simulink library "tqr"  (R2021b)
settings: Solver=VariableStepAuto  StartTime=0.0  StopTime=10.0  RelTol=1e-3
undefined symbols (not defined in the file or in its folder): ATQR_AltRDCActiveFEDUInc_X_pct, ATQR_AltRDCActiveFEDUInc_Y_enum, ATQR_AltRDCActiveFEDUTs_X_pct, ATQR_AltRDCActiveFEDUTs_Y_enum, ATQR_AltRDCActiveREDUInc_X_pct, ATQR_AltRDCActiveREDUInc_Y_enum, ATQR_AltRDCActiveREDUTs_X_pct, ATQR_AltRDCActiveREDUTs_Y_enum, ATQR_CreepFEDUTqIncSR_X_rpm, ATQR_CreepFEDUTqIncSR_Y_Nm, ATQR_CreepFEDUTs_X_rpm, ATQR_CreepFEDUTs_Y_Nm, ATQR_EcoTqFrIncGain_X_Nm, ATQR_EcoTqFrIncGain_Y_pct, ATQR_EcoTqRrIncGain_X_Nm, ATQR_EcoTqRrIncGain_Y_pct, ATQR_EL1FEDUTqDecSR_Y_Nm, ATQR_EL1FEDUTqIncSR_X_rpm, ATQR_EL1FEDUTqIncSR_Y_pct, ATQR_EL1FEDUTs_X_rpm, ATQR_EL1FEDUTs_Y_Nm, ATQR_EL1REDUTqDecSR_Y_Nm, ATQR_EL1REDUTs_Y_Nm, ATQR_FEDUEL1RegenTs_X_rpm, ATQR_FEDUTIPOutTs_X_rpm, ATQR_FrNegRateLimitIncN_X_rpm, ATQR_FrNegRateLimitIncN_Y_Nm, ATQR_FrPosRateLimitIncN_X_rpm, ATQR_FrPosRateLimitIncN_Y_Nm, ATQR_FShaftSpdTqLimCoe_X_rpm, ATQR_FTimerTqLimCoe_X_s, ATQR_FTqZeroTransUpBoundN_X_rpm, ATQR_NL1FEDUTqDecSR_Y_Nm, ATQR_NL1FEDUTqIncSR_X_rpm, ATQR_NL1FEDUTqIncSR_Y_pct, ATQR_NL1FEDUTs_X_rpm, ATQR_NL1FEDUTs_Y_Nm, ATQR_NL1REDUTqDecSR_Y_Nm, ATQR_NL1REDUTs_Y_Nm, ATQR_NormalTqFrIncGain_X_Nm, ATQR_NormalTqFrIncGain_Y_pct, ATQR_NormalTqRrIncGain_X_Nm, ATQR_NormalTqRrIncGain_Y_pct, ATQR_RrNegRateLimitIncN_X_rpm, ATQR_RrNegRateLimitIncN_Y_Nm, ATQR_RrPosRateLimitIncN_X_rpm, ATQR_RrPosRateLimitIncN_Y_Nm, ATQR_RShaftSpdTqLimCoe_X_rpm, ATQR_RTimerTqLimCoe_X_s, ATQR_SL1FEDUTqDecSR_Y_Nm, ATQR_SL1FEDUTqIncSR_X_rpm, ATQR_SL1FEDUTqIncSR_Y_pct, ATQR_SL1FEDUTs_X_rpm, ATQR_SL1FEDUTs_Y_Nm, ATQR_SL1REDUTqDecSR_Y_Nm, ATQR_SL1REDUTs_Y_Nm, ATQR_SportTqFrIncGain_X_Nm, ATQR_SportTqFrIncGain_Y_pct, ATQR_SportTqRrIncGain_X_Nm, ATQR_SportTqRrIncGain_Y_pct ... (+261)
libraries: hcu_lib x14, simulink x12, $bdroot x3
(part 7 of 9)

== system tqr/TQR/Determine Torque Request/TorqueArbitrament/TorqueSmooth/Front First order filter input tau map and determination/VTQR_SPORTFEDUTs_c/Invalid ==
  VTQR_FEDUWhlTqReqSmoothDelay_Nm : Inport
  VTQD_TqTargetShaftSpd_rpm : Inport  Port=2
  Action Port : ActionPort
  MTQR_SL1FEDUTs_Z_c : Lookup_n-D  BreakpointsForDimension1=ATQR_SL1FEDUTs_Y_Nm  BreakpointsForDimension2=ATQR_SL1FEDUTs_X_rpm  Table=MTQR_SL1FEDUTs_Z_c  ExtrapMethod=Clip  InternalRulePriority=Speed  RndMeth=Simplest  InputSameDT=on
      settings: InputPortMap=u0,u1
  VTQR_SL1FEDUTs_c : Outport
  wires:
  VTQR_FEDUWhlTqReqSmoothDelay_Nm/1 -> MTQR_SL1FEDUTs_Z_c/1
  VTQD_TqTargetShaftSpd_rpm/1 -> MTQR_SL1FEDUTs_Z_c/2
  MTQR_SL1FEDUTs_Z_c/1 -> VTQR_SL1FEDUTs_c/1

== system tqr/TQR/Determine Torque Request/TorqueArbitrament/TorqueSmooth/Front First order filter input tau map and determination/VTQR_SPORTFEDUTs_c/LV1 ==
  VTQR_FEDUWhlTqReqSmoothDelay_Nm : Inport
  VTQD_TqTargetShaftSpd_rpm : Inport  Port=2
  Action Port : ActionPort
  MTQR_SL1FEDUTs_Z_c : Lookup_n-D  BreakpointsForDimension1=ATQR_SL1FEDUTs_Y_Nm  BreakpointsForDimension2=ATQR_SL1FEDUTs_X_rpm  Table=MTQR_SL1FEDUTs_Z_c  ExtrapMethod=Clip  InternalRulePriority=Speed  RndMeth=Simplest  InputSameDT=on
      settings: InputPortMap=u0,u1
  VTQR_SL1FEDUTs_c : Outport
  wires:
  MTQR_SL1FEDUTs_Z_c/1 -> VTQR_SL1FEDUTs_c/1
  VTQD_TqTargetShaftSpd_rpm/1 -> MTQR_SL1FEDUTs_Z_c/2
  VTQR_FEDUWhlTqReqSmoothDelay_Nm/1 -> MTQR_SL1FEDUTs_Z_c/1

== system tqr/TQR/Determine Torque Request/TorqueArbitrament/TorqueSmooth/Front First order filter input tau map and determination/VTQR_SPORTFEDUTs_c/LV2 ==
  VTQR_FEDUWhlTqReqSmoothDelay_Nm : Inport
  VTQD_TqTargetShaftSpd_rpm : Inport  Port=2
  Action Port : ActionPort
  MTQR_SL2FEDUTs_Z_c : Lookup_n-D  BreakpointsForDimension1=ATQR_SL1FEDUTs_Y_Nm  BreakpointsForDimension2=ATQR_SL1FEDUTs_X_rpm  Table=MTQR_SL2FEDUTs_Z_c  ExtrapMethod=Clip  InternalRulePriority=Speed  RndMeth=Simplest  InputSameDT=on
      settings: InputPortMap=u0,u1
  VTQR_SL2FEDUTs_c : Outport
  wires:
  VTQR_FEDUWhlTqReqSmoothDelay_Nm/1 -> MTQR_SL2FEDUTs_Z_c/1
  VTQD_TqTargetShaftSpd_rpm/1 -> MTQR_SL2FEDUTs_Z_c/2
  MTQR_SL2FEDUTs_Z_c/1 -> VTQR_SL2FEDUTs_c/1

== system tqr/TQR/Determine Torque Request/TorqueArbitrament/TorqueSmooth/Front First order filter input tau map and determination/VTQR_SPORTFEDUTs_c/LV3 ==
  VTQR_FEDUWhlTqReqSmoothDelay_Nm : Inport
  VTQD_TqTargetShaftSpd_rpm : Inport  Port=2
  Action Port : ActionPort
  MTQR_SL3FEDUTs_Z_c : Lookup_n-D  BreakpointsForDimension1=ATQR_SL1FEDUTs_Y_Nm  BreakpointsForDimension2=ATQR_SL1FEDUTs_X_rpm  Table=MTQR_SL3FEDUTs_Z_c  ExtrapMethod=Clip  InternalRulePriority=Speed  RndMeth=Simplest  InputSameDT=on
      settings: InputPortMap=u0,u1
  VTQR_SL3FEDUTs_c : Outport
  wires:
  VTQR_FEDUWhlTqReqSmoothDelay_Nm/1 -> MTQR_SL3FEDUTs_Z_c/1
  VTQD_TqTargetShaftSpd_rpm/1 -> MTQR_SL3FEDUTs_Z_c/2
  MTQR_SL3FEDUTs_Z_c/1 -> VTQR_SL3FEDUTs_c/1

== system tqr/TQR/Determine Torque Request/TorqueArbitrament/TorqueSmooth/Front First order filter input tau map and determination/VTQR_SPORTFEDUTs_c/LV4 ==
  VTQR_FEDUWhlTqReqSmoothDelay_Nm : Inport
  VTQD_TqTargetShaftSpd_rpm : Inport  Port=2
  Action Port : ActionPort
  MTQR_SL4FEDUTs_Z_c : Lookup_n-D  BreakpointsForDimension1=ATQR_SL1FEDUTs_Y_Nm  BreakpointsForDimension2=ATQR_SL1FEDUTs_X_rpm  Table=MTQR_SL4FEDUTs_Z_c  ExtrapMethod=Clip  InternalRulePriority=Speed  RndMeth=Simplest  InputSameDT=on
      settings: InputPortMap=u0,u1
  VTQR_SL4FEDUTs_c : Outport
  wires:
  VTQR_FEDUWhlTqReqSmoothDelay_Nm/1 -> MTQR_SL4FEDUTs_Z_c/1
  VTQD_TqTargetShaftSpd_rpm/1 -> MTQR_SL4FEDUTs_Z_c/2
  MTQR_SL4FEDUTs_Z_c/1 -> VTQR_SL4FEDUTs_c/1

== system tqr/TQR/Determine Torque Request/TorqueArbitrament/TorqueSmooth/Front First order filter input tau map and determination/VTQR_SPORTFEDUTs_c/LV5 ==
  VTQR_FEDUWhlTqReqSmoothDelay_Nm : Inport
  VTQD_TqTargetShaftSpd_rpm : Inport  Port=2
  Action Port : ActionPort
  MTQR_SL5FEDUTs_Z_c : Lookup_n-D  BreakpointsForDimension1=ATQR_SL1FEDUTs_Y_Nm  BreakpointsForDimension2=ATQR_SL1FEDUTs_X_rpm  Table=MTQR_SL5FEDUTs_Z_c  ExtrapMethod=Clip  InternalRulePriority=Speed  RndMeth=Simplest  InputSameDT=on
      settings: InputPortMap=u0,u1
  VTQR_SL5FEDUTs_c : Outport
  wires:
  VTQR_FEDUWhlTqReqSmoothDelay_Nm/1 -> MTQR_SL5FEDUTs_Z_c/1
  VTQD_TqTargetShaftSpd_rpm/1 -> MTQR_SL5FEDUTs_Z_c/2
  MTQR_SL5FEDUTs_Z_c/1 -> VTQR_SL5FEDUTs_c/1

== system tqr/TQR/Determine Torque Request/TorqueArbitrament/TorqueSmooth/Front First order filter input tau map and determination/VTQR_SPORTFEDUTs_c/OPD ==
  VTQR_FEDUWhlTqReqSmoothDelay_Nm : Inport
  VTQD_TqTargetShaftSpd_rpm : Inport  Port=2
  Action Port : ActionPort
  MTQR_SOPDFEDUTs_Z_c : Lookup_n-D  BreakpointsForDimension1=ATQR_SL1FEDUTs_Y_Nm  BreakpointsForDimension2=ATQR_SL1FEDUTs_X_rpm  Table=MTQR_SOPDFEDUTs_Z_c  ExtrapMethod=Clip  InternalRulePriority=Speed  RndMeth=Simplest  InputSameDT=on
      settings: InputPortMap=u0,u1
  VTQR_SOPDFEDUTs_c : Outport
  wires:
  VTQR_FEDUWhlTqReqSmoothDelay_Nm/1 -> MTQR_SOPDFEDUTs_Z_c/1
  VTQD_TqTargetShaftSpd_rpm/1 -> MTQR_SOPDFEDUTs_Z_c/2
  MTQR_SOPDFEDUTs_Z_c/1 -> VTQR_SOPDFEDUTs_c/1

== system tqr/TQR/Determine Torque Request/TorqueArbitrament/TorqueSmooth/Front wheel rate limit determination/Negative Rate limit Determination/VTQR_FrNegRateLimitDecE_Nm ==
  VTQD_TqTargetShaftSpd_rpm : Inport
  VTQR_FEDUWhlTqReqSmoothDelay_Nm : Inport  Port=2
  Action Port : ActionPort
  MTQR_FrNegRateLimitDecE_Z_Nm : Lookup_n-D  BreakpointsForDimension1=ATQR_FrNegRateLimitIncN_Y_Nm  BreakpointsForDimension2=ATQR_FrNegRateLimitIncN_X_rpm  Table=MTQR_FrNegRateLimitDecE_Z_Nm  ExtrapMethod=Clip  UseLastTableValue=on  InternalRulePriority=Speed  RndMeth=Simplest  InputSameDT=on
      settings: InputPortMap=u0,u1
  VTQR_FrNegRateLimitDecE_Nm : Outport
  wires:
  MTQR_FrNegRateLimitDecE_Z_Nm/1 -> VTQR_FrNegRateLimitDecE_Nm/1  "VTQR_FrNegRateLimitDecE_Nm"
  VTQR_FEDUWhlTqReqSmoothDelay_Nm/1 -> MTQR_FrNegRateLimitDecE_Z_Nm/1
  VTQD_TqTargetShaftSpd_rpm/1 -> MTQR_FrNegRateLimitDecE_Z_Nm/2

== system tqr/TQR/Determine Torque Request/TorqueArbitrament/TorqueSmooth/Front wheel rate limit determination/Negative Rate limit Determination/VTQR_FrNegRateLimitDecN_Nm ==
  VTQD_TqTargetShaftSpd_rpm : Inport
  VTQR_FEDUWhlTqReqSmoothDelay_Nm : Inport  Port=2
  Action Port : ActionPort
  MTQR_FrNegRateLimitDecN_Z_Nm : Lookup_n-D  BreakpointsForDimension1=ATQR_FrNegRateLimitIncN_Y_Nm  BreakpointsForDimension2=ATQR_FrNegRateLimitIncN_X_rpm  Table=MTQR_FrNegRateLimitDecN_Z_Nm  ExtrapMethod=Clip  UseLastTableValue=on  InternalRulePriority=Speed  RndMeth=Simplest  InputSameDT=on
      settings: InputPortMap=u0,u1
  VTQR_FrNegRateLimitDecN_Nm : Outport
  wires:
  MTQR_FrNegRateLimitDecN_Z_Nm/1 -> VTQR_FrNegRateLimitDecN_Nm/1  "VTQR_FrNegRateLimitDecN_Nm"
  VTQR_FEDUWhlTqReqSmoothDelay_Nm/1 -> MTQR_FrNegRateLimitDecN_Z_Nm/1
  VTQD_TqTargetShaftSpd_rpm/1 -> MTQR_FrNegRateLimitDecN_Z_Nm/2

== system tqr/TQR/Determine Torque Request/TorqueArbitrament/TorqueSmooth/Front wheel rate limit determination/Negative Rate limit Determination/VTQR_FrNegRateLimitDecS_Nm ==
  VTQD_TqTargetShaftSpd_rpm : Inport
  VTQR_FEDUWhlTqReqSmoothDelay_Nm : Inport  Port=2
  Action Port : ActionPort
  MTQR_FrNegRateLimitDecS_Z_Nm : Lookup_n-D  BreakpointsForDimension1=ATQR_FrNegRateLimitIncN_Y_Nm  BreakpointsForDimension2=ATQR_FrNegRateLimitIncN_X_rpm  Table=MTQR_FrNegRateLimitDecS_Z_Nm  ExtrapMethod=Clip  UseLastTableValue=on  InternalRulePriority=Speed  RndMeth=Simplest  InputSameDT=on
      settings: InputPortMap=u0,u1
  VTQR_FrNegRateLimitDecS_Nm : Outport
  wires:
  MTQR_FrNegRateLimitDecS_Z_Nm/1 -> VTQR_FrNegRateLimitDecS_Nm/1  "VTQR_FrNegRateLimitDecS_Nm"
  VTQD_TqTargetShaftSpd_rpm/1 -> MTQR_FrNegRateLimitDecS_Z_Nm/2
  VTQR_FEDUWhlTqReqSmoothDelay_Nm/1 -> MTQR_FrNegRateLimitDecS_Z_Nm/1

== system tqr/TQR/Determine Torque Request/TorqueArbitrament/TorqueSmooth/Front wheel rate limit determination/Negative Rate limit Determination/VTQR_FrNegRateLimitIncE_Nm ==
  VTQD_TqTargetShaftSpd_rpm : Inport
  VTQR_FEDUWhlTqReqSmoothDelay_Nm : Inport  Port=2
  Action Port : ActionPort
  MTQR_FrNegRateLimitIncE_Z_Nm : Lookup_n-D  BreakpointsForDimension1=ATQR_FrNegRateLimitIncN_Y_Nm  BreakpointsForDimension2=ATQR_FrNegRateLimitIncN_X_rpm  Table=MTQR_FrNegRateLimitIncE_Z_Nm  ExtrapMethod=Clip  UseLastTableValue=on  InternalRulePriority=Speed  RndMeth=Simplest  InputSameDT=on
      settings: InputPortMap=u0,u1
  VTQR_FrNegRateLimitIncE_Nm : Outport
  wires:
  MTQR_FrNegRateLimitIncE_Z_Nm/1 -> VTQR_FrNegRateLimitIncE_Nm/1  "VTQR_FrNegRateLimitIncE_Nm"
  VTQR_FEDUWhlTqReqSmoothDelay_Nm/1 -> MTQR_FrNegRateLimitIncE_Z_Nm/1
  VTQD_TqTargetShaftSpd_rpm/1 -> MTQR_FrNegRateLimitIncE_Z_Nm/2

== system tqr/TQR/Determine Torque Request/TorqueArbitrament/TorqueSmooth/Front wheel rate limit determination/Negative Rate limit Determination/VTQR_FrNegRateLimitIncN_Nm ==
  VTQD_TqTargetShaftSpd_rpm : Inport
  VTQR_FEDUWhlTqReqSmoothDelay_Nm : Inport  Port=2
  Action Port : ActionPort
  MTQR_FrNegRateLimitIncN_Z_Nm : Lookup_n-D  BreakpointsForDimension1=ATQR_FrNegRateLimitIncN_Y_Nm  BreakpointsForDimension2=ATQR_FrNegRateLimitIncN_X_rpm  Table=MTQR_FrNegRateLimitIncN_Z_Nm  ExtrapMethod=Clip  UseLastTableValue=on  InternalRulePriority=Speed  RndMeth=Simplest  InputSameDT=on
      settings: InputPortMap=u0,u1
  VTQR_FrNegRateLimitIncN_Nm : Outport
  wires:
  MTQR_FrNegRateLimitIncN_Z_Nm/1 -> VTQR_FrNegRateLimitIncN_Nm/1  "VTQR_FrNegRateLimitIncN_Nm"
  VTQR_FEDUWhlTqReqSmoothDelay_Nm/1 -> MTQR_FrNegRateLimitIncN_Z_Nm/1
  VTQD_TqTargetShaftSpd_rpm/1 -> MTQR_FrNegRateLimitIncN_Z_Nm/2

== system tqr/TQR/Determine Torque Request/TorqueArbitrament/TorqueSmooth/Front wheel rate limit determination/Negative Rate limit Determination/VTQR_FrNegRateLimitIncS_Nm ==
  VTQD_TqTargetShaftSpd_rpm : Inport
  VTQR_FEDUWhlTqReqSmoothDelay_Nm : Inport  Port=2
  Action Port : ActionPort
  MTQR_FrNegRateLimitIncS_Z_Nm : Lookup_n-D  BreakpointsForDimension1=ATQR_FrNegRateLimitIncN_Y_Nm  BreakpointsForDimension2=ATQR_FrNegRateLimitIncN_X_rpm  Table=MTQR_FrNegRateLimitIncS_Z_Nm  ExtrapMethod=Clip  UseLastTableValue=on  InternalRulePriority=Speed  RndMeth=Simplest  InputSameDT=on
      settings: InputPortMap=u0,u1
  VTQR_FrNegRateLimitIncS_Nm : Outport
  wires:
  MTQR_FrNegRateLimitIncS_Z_Nm/1 -> VTQR_FrNegRateLimitIncS_Nm/1  "VTQR_FrNegRateLimitIncS_Nm"
  VTQD_TqTargetShaftSpd_rpm/1 -> MTQR_FrNegRateLimitIncS_Z_Nm/2
  VTQR_FEDUWhlTqReqSmoothDelay_Nm/1 -> MTQR_FrNegRateLimitIncS_Z_Nm/1

== system tqr/TQR/Determine Torque Request/TorqueArbitrament/TorqueSmooth/Front wheel rate limit determination/Positive Rate limit Determination/VTQR_FrPosRateLimitDecE_Nm ==
  VTQD_TqTargetShaftSpd_rpm : Inport
  VTQR_FEDUWhlTqReqSmoothDelay_Nm : Inport  Port=2
  Action Port : ActionPort
  MTQR_FrPosRateLimitDecE_Z_Nm : Lookup_n-D  BreakpointsForDimension1=ATQR_FrPosRateLimitIncN_Y_Nm  BreakpointsForDimension2=ATQR_FrPosRateLimitIncN_X_rpm  Table=MTQR_FrPosRateLimitDecE_Z_Nm  ExtrapMethod=Clip  UseLastTableValue=on  InternalRulePriority=Speed  RndMeth=Simplest  InputSameDT=on
      settings: InputPortMap=u0,u1
  VTQR_FrPosRateLimitDecE_Nm : Outport
  wires:
  VTQD_TqTargetShaftSpd_rpm/1 -> MTQR_FrPosRateLimitDecE_Z_Nm/2
  VTQR_FEDUWhlTqReqSmoothDelay_Nm/1 -> MTQR_FrPosRateLimitDecE_Z_Nm/1
  MTQR_FrPosRateLimitDecE_Z_Nm/1 -> VTQR_FrPosRateLimitDecE_Nm/1  "VTQR_FrPosRateLimitDecE_Nm"

== system tqr/TQR/Determine Torque Request/TorqueArbitrament/TorqueSmooth/Front wheel rate limit determination/Positive Rate limit Determination/VTQR_FrPosRateLimitDecN_Nm ==
  VTQD_TqTargetShaftSpd_rpm : Inport
  VTQR_FEDUWhlTqReqSmoothDelay_Nm : Inport  Port=2
  Action Port : ActionPort
  MTQR_FrPosRateLimitDecN_Z_Nm : Lookup_n-D  BreakpointsForDimension1=ATQR_FrPosRateLimitIncN_Y_Nm  BreakpointsForDimension2=ATQR_FrPosRateLimitIncN_X_rpm  Table=MTQR_FrPosRateLimitDecN_Z_Nm  ExtrapMethod=Clip  UseLastTableValue=on  InternalRulePriority=Speed  RndMeth=Simplest  InputSameDT=on
      settings: InputPortMap=u0,u1
  VTQR_FrPosRateLimitDecN_Nm : Outport
  wires:
  VTQD_TqTargetShaftSpd_rpm/1 -> MTQR_FrPosRateLimitDecN_Z_Nm/2
  VTQR_FEDUWhlTqReqSmoothDelay_Nm/1 -> MTQR_FrPosRateLimitDecN_Z_Nm/1
  MTQR_FrPosRateLimitDecN_Z_Nm/1 -> VTQR_FrPosRateLimitDecN_Nm/1  "VTQR_FrPosRateLimitDecN_Nm"

== system tqr/TQR/Determine Torque Request/TorqueArbitrament/TorqueSmooth/Front wheel rate limit determination/Positive Rate limit Determination/VTQR_FrPosRateLimitDecS_Nm ==
  VTQD_TqTargetShaftSpd_rpm : Inport
  VTQR_FEDUWhlTqReqSmoothDelay_Nm : Inport  Port=2
  Action Port : ActionPort
  MTQR_FrPosRateLimitDecS_Z_Nm : Lookup_n-D  BreakpointsForDimension1=ATQR_FrPosRateLimitIncN_Y_Nm  BreakpointsForDimension2=ATQR_FrPosRateLimitIncN_X_rpm  Table=MTQR_FrPosRateLimitDecS_Z_Nm  ExtrapMethod=Clip  UseLastTableValue=on  InternalRulePriority=Speed  RndMeth=Simplest  InputSameDT=on
      settings: InputPortMap=u0,u1
  VTQR_FrPosRateLimitDecS_Nm : Outport
  wires:
  VTQR_FEDUWhlTqReqSmoothDelay_Nm/1 -> MTQR_FrPosRateLimitDecS_Z_Nm/1
  VTQD_TqTargetShaftSpd_rpm/1 -> MTQR_FrPosRateLimitDecS_Z_Nm/2
  MTQR_FrPosRateLimitDecS_Z_Nm/1 -> VTQR_FrPosRateLimitDecS_Nm/1  "VTQR_FrPosRateLimitDecS_Nm"

== system tqr/TQR/Determine Torque Request/TorqueArbitrament/TorqueSmooth/Front wheel rate limit determination/Positive Rate limit Determination/VTQR_FrPosRateLimitIncE_Nm ==
  VTQD_TqTargetShaftSpd_rpm : Inport
  VTQR_FEDUWhlTqReqSmoothDelay_Nm : Inport  Port=2
  Action Port : ActionPort
  MTQR_FrPosRateLimitIncE_Z_Nm : Lookup_n-D  BreakpointsForDimension1=ATQR_FrPosRateLimitIncN_Y_Nm  BreakpointsForDimension2=ATQR_FrPosRateLimitIncN_X_rpm  Table=MTQR_FrPosRateLimitIncE_Z_Nm  ExtrapMethod=Clip  UseLastTableValue=on  InternalRulePriority=Speed  RndMeth=Simplest  InputSameDT=on
      settings: InputPortMap=u0,u1
  VTQR_FrPosRateLimitIncE_Nm : Outport
  wires:
  VTQD_TqTargetShaftSpd_rpm/1 -> MTQR_FrPosRateLimitIncE_Z_Nm/2
  VTQR_FEDUWhlTqReqSmoothDelay_Nm/1 -> MTQR_FrPosRateLimitIncE_Z_Nm/1
  MTQR_FrPosRateLimitIncE_Z_Nm/1 -> VTQR_FrPosRateLimitIncE_Nm/1  "VTQR_FrPosRateLimitIncE_Nm"

== system tqr/TQR/Determine Torque Request/TorqueArbitrament/TorqueSmooth/Front wheel rate limit determination/Positive Rate limit Determination/VTQR_FrPosRateLimitIncN_Nm ==
  VTQD_TqTargetShaftSpd_rpm : Inport
  VTQR_FEDUWhlTqReqSmoothDelay_Nm : Inport  Port=2
  Action Port : ActionPort
  MTQR_FrPosRateLimitIncN_Z_Nm : Lookup_n-D  BreakpointsForDimension1=ATQR_FrPosRateLimitIncN_Y_Nm  BreakpointsForDimension2=ATQR_FrPosRateLimitIncN_X_rpm  Table=MTQR_FrPosRateLimitIncN_Z_Nm  ExtrapMethod=Clip  UseLastTableValue=on  InternalRulePriority=Speed  RndMeth=Simplest  InputSameDT=on
      settings: InputPortMap=u0,u1
  VTQR_FrPosRateLimitIncN_Nm : Outport
  wires:
  VTQD_TqTargetShaftSpd_rpm/1 -> MTQR_FrPosRateLimitIncN_Z_Nm/2
  VTQR_FEDUWhlTqReqSmoothDelay_Nm/1 -> MTQR_FrPosRateLimitIncN_Z_Nm/1
  MTQR_FrPosRateLimitIncN_Z_Nm/1 -> VTQR_FrPosRateLimitIncN_Nm/1  "VTQR_FrPosRateLimitIncN_Nm"

== system tqr/TQR/Determine Torque Request/TorqueArbitrament/TorqueSmooth/Front wheel rate limit determination/Positive Rate limit Determination/VTQR_FrPosRateLimitIncS_Nm ==
  VTQD_TqTargetShaftSpd_rpm : Inport
  VTQR_FEDUWhlTqReqSmoothDelay_Nm : Inport  Port=2
  Action Port : ActionPort
  MTQR_FrPosRateLimitIncS_Z_Nm : Lookup_n-D  BreakpointsForDimension1=ATQR_FrPosRateLimitIncN_Y_Nm  BreakpointsForDimension2=ATQR_FrPosRateLimitIncN_X_rpm  Table=MTQR_FrPosRateLimitIncS_Z_Nm  ExtrapMethod=Clip  UseLastTableValue=on  InternalRulePriority=Speed  RndMeth=Simplest  InputSameDT=on
      settings: InputPortMap=u0,u1
  VTQR_FrPosRateLimitIncS_Nm : Outport
  wires:
  VTQR_FEDUWhlTqReqSmoothDelay_Nm/1 -> MTQR_FrPosRateLimitIncS_Z_Nm/1
  VTQD_TqTargetShaftSpd_rpm/1 -> MTQR_FrPosRateLimitIncS_Z_Nm/2
  MTQR_FrPosRateLimitIncS_Z_Nm/1 -> VTQR_FrPosRateLimitIncS_Nm/1  "VTQR_FrPosRateLimitIncS_Nm"

== system tqr/TQR/Determine Torque Request/TorqueArbitrament/TorqueSmooth/Front wheel rate limit determination/VTQR_ECOFEDURateLimitDec_Nm/Invalid ==
  VTQR_FEDUWhlTqReqSmoothDelay_Nm : Inport
  VTQD_TqTargetShaftSpd_rpm : Inport  Port=2
  Action Port : ActionPort
  MTQR_EL1FEDUTqDecSR_Z_Nm : Lookup_n-D  BreakpointsForDimension1=ATQR_EL1FEDUTqDecSR_Y_Nm  BreakpointsForDimension2=ATQR_EL1FEDUTqIncSR_X_rpm  Table=MTQR_EL1FEDUTqDecSR_Z_Nm  ExtrapMethod=Clip  InternalRulePriority=Speed  RndMeth=Simplest  InputSameDT=on
      settings: InputPortMap=u0,u1
  VTQR_EL1FEDUTqDecSR_Nm : Outport
  wires:
  VTQD_TqTargetShaftSpd_rpm/1 -> MTQR_EL1FEDUTqDecSR_Z_Nm/2
  MTQR_EL1FEDUTqDecSR_Z_Nm/1 -> VTQR_EL1FEDUTqDecSR_Nm/1
  VTQR_FEDUWhlTqReqSmoothDelay_Nm/1 -> MTQR_EL1FEDUTqDecSR_Z_Nm/1

== system tqr/TQR/Determine Torque Request/TorqueArbitrament/TorqueSmooth/Front wheel rate limit determination/VTQR_ECOFEDURateLimitDec_Nm/LV1 ==
  VTQR_FEDUWhlTqReqSmoothDelay_Nm : Inport
  VTQD_TqTargetShaftSpd_rpm : Inport  Port=2
  Action Port : ActionPort
  MTQR_EL1FEDUTqDecSR_Z_Nm : Lookup_n-D  BreakpointsForDimension1=ATQR_EL1FEDUTqDecSR_Y_Nm  BreakpointsForDimension2=ATQR_EL1FEDUTqIncSR_X_rpm  Table=MTQR_EL1FEDUTqDecSR_Z_Nm  ExtrapMethod=Clip  InternalRulePriority=Speed  RndMeth=Simplest  InputSameDT=on
      settings: InputPortMap=u0,u1
  VTQR_EL1FEDUTqDecSR_Nm : Outport
  wires:
  VTQR_FEDUWhlTqReqSmoothDelay_Nm/1 -> MTQR_EL1FEDUTqDecSR_Z_Nm/1
  MTQR_EL1FEDUTqDecSR_Z_Nm/1 -> VTQR_EL1FEDUTqDecSR_Nm/1
  VTQD_TqTargetShaftSpd_rpm/1 -> MTQR_EL1FEDUTqDecSR_Z_Nm/2

== system tqr/TQR/Determine Torque Request/TorqueArbitrament/TorqueSmooth/Front wheel rate limit determination/VTQR_ECOFEDURateLimitDec_Nm/LV2 ==
  VTQR_FEDUWhlTqReqSmoothDelay_Nm : Inport
  VTQD_TqTargetShaftSpd_rpm : Inport  Port=2
  Action Port : ActionPort
  MTQR_EL2FEDUTqDecSR_Z_Nm : Lookup_n-D  BreakpointsForDimension1=ATQR_EL1FEDUTqDecSR_Y_Nm  BreakpointsForDimension2=ATQR_EL1FEDUTqIncSR_X_rpm  Table=MTQR_EL2FEDUTqDecSR_Z_Nm  ExtrapMethod=Clip  InternalRulePriority=Speed  RndMeth=Simplest  InputSameDT=on
      settings: InputPortMap=u0,u1
  VTQR_EL2FEDUTqDecSR_Nm : Outport
  wires:
  MTQR_EL2FEDUTqDecSR_Z_Nm/1 -> VTQR_EL2FEDUTqDecSR_Nm/1
  VTQR_FEDUWhlTqReqSmoothDelay_Nm/1 -> MTQR_EL2FEDUTqDecSR_Z_Nm/1
  VTQD_TqTargetShaftSpd_rpm/1 -> MTQR_EL2FEDUTqDecSR_Z_Nm/2

== system tqr/TQR/Determine Torque Request/TorqueArbitrament/TorqueSmooth/Front wheel rate limit determination/VTQR_ECOFEDURateLimitDec_Nm/LV3 ==
  VTQR_FEDUWhlTqReqSmoothDelay_Nm : Inport
  VTQD_TqTargetShaftSpd_rpm : Inport  Port=2
  Action Port : ActionPort
  MTQR_EL3FEDUTqDecSR_Z_Nm : Lookup_n-D  BreakpointsForDimension1=ATQR_EL1FEDUTqDecSR_Y_Nm  BreakpointsForDimension2=ATQR_EL1FEDUTqIncSR_X_rpm  Table=MTQR_EL3FEDUTqDecSR_Z_Nm  ExtrapMethod=Clip  InternalRulePriority=Speed  RndMeth=Simplest  InputSameDT=on
      settings: InputPortMap=u0,u1
  VTQR_EL3FEDUTqDecSR_Nm : Outport
  wires:
  VTQR_FEDUWhlTqReqSmoothDelay_Nm/1 -> MTQR_EL3FEDUTqDecSR_Z_Nm/1
  VTQD_TqTargetShaftSpd_rpm/1 -> MTQR_EL3FEDUTqDecSR_Z_Nm/2
  MTQR_EL3FEDUTqDecSR_Z_Nm/1 -> VTQR_EL3FEDUTqDecSR_Nm/1

== system tqr/TQR/Determine Torque Request/TorqueArbitrament/TorqueSmooth/Front wheel rate limit determination/VTQR_ECOFEDURateLimitDec_Nm/LV4 ==
  VTQR_FEDUWhlTqReqSmoothDelay_Nm : Inport
  VTQD_TqTargetShaftSpd_rpm : Inport  Port=2
  Action Port : ActionPort
  MTQR_EL4FEDUTqDecSR_Z_Nm : Lookup_n-D  BreakpointsForDimension1=ATQR_EL1FEDUTqDecSR_Y_Nm  BreakpointsForDimension2=ATQR_EL1FEDUTqIncSR_X_rpm  Table=MTQR_EL4FEDUTqDecSR_Z_Nm  ExtrapMethod=Clip  InternalRulePriority=Speed  RndMeth=Simplest  InputSameDT=on
      settings: InputPortMap=u0,u1
  VTQR_EL4FEDUTqDecSR_Nm : Outport
  wires:
  VTQR_FEDUWhlTqReqSmoothDelay_Nm/1 -> MTQR_EL4FEDUTqDecSR_Z_Nm/1
  VTQD_TqTargetShaftSpd_rpm/1 -> MTQR_EL4FEDUTqDecSR_Z_Nm/2
  MTQR_EL4FEDUTqDecSR_Z_Nm/1 -> VTQR_EL4FEDUTqDecSR_Nm/1

== system tqr/TQR/Determine Torque Request/TorqueArbitrament/TorqueSmooth/Front wheel rate limit determination/VTQR_ECOFEDURateLimitDec_Nm/LV5 ==
  VTQR_FEDUWhlTqReqSmoothDelay_Nm : Inport
  VTQD_TqTargetShaftSpd_rpm : Inport  Port=2
  Action Port : ActionPort
  MTQR_EL5FEDUTqDecSR_Z_Nm : Lookup_n-D  BreakpointsForDimension1=ATQR_EL1FEDUTqDecSR_Y_Nm  BreakpointsForDimension2=ATQR_EL1FEDUTqIncSR_X_rpm  Table=MTQR_EL5FEDUTqDecSR_Z_Nm  ExtrapMethod=Clip  InternalRulePriority=Speed  RndMeth=Simplest  InputSameDT=on
      settings: InputPortMap=u0,u1
  VTQR_EL5FEDUTqIDecSR_Nm : Outport
  wires:
  VTQR_FEDUWhlTqReqSmoothDelay_Nm/1 -> MTQR_EL5FEDUTqDecSR_Z_Nm/1
  VTQD_TqTargetShaftSpd_rpm/1 -> MTQR_EL5FEDUTqDecSR_Z_Nm/2
  MTQR_EL5FEDUTqDecSR_Z_Nm/1 -> VTQR_EL5FEDUTqIDecSR_Nm/1

== system tqr/TQR/Determine Torque Request/TorqueArbitrament/TorqueSmooth/Front wheel rate limit determination/VTQR_ECOFEDURateLimitDec_Nm/OPD ==
  VTQR_FEDUWhlTqReqSmoothDelay_Nm : Inport
  VTQD_TqTargetShaftSpd_rpm : Inport  Port=2
  Action Port : ActionPort
  MTQR_EOPDFEDUTqDecSR_Z_Nm : Lookup_n-D  BreakpointsForDimension1=ATQR_EL1FEDUTqDecSR_Y_Nm  BreakpointsForDimension2=ATQR_EL1FEDUTqIncSR_X_rpm  Table=MTQR_EOPDFEDUTqDecSR_Z_Nm  ExtrapMethod=Clip  InternalRulePriority=Speed  RndMeth=Simplest  InputSameDT=on
      settings: InputPortMap=u0,u1
  VTQR_EOPDFEDUTqDecSR_Nm : Outport
  wires:
  VTQR_FEDUWhlTqReqSmoothDelay_Nm/1 -> MTQR_EOPDFEDUTqDecSR_Z_Nm/1
  VTQD_TqTargetShaftSpd_rpm/1 -> MTQR_EOPDFEDUTqDecSR_Z_Nm/2
  MTQR_EOPDFEDUTqDecSR_Z_Nm/1 -> VTQR_EOPDFEDUTqDecSR_Nm/1

== system tqr/TQR/Determine Torque Request/TorqueArbitrament/TorqueSmooth/Front wheel rate limit determination/VTQR_ECOFEDURateLimitInc_Nm/Invalid ==
  VDHP_ActAPSPosn_pct : Inport
  VTQD_TqTargetShaftSpd_rpm : Inport  Port=2
  Action Port : ActionPort
  MTQR_EL1FEDUTqIncSR_Z_Nm : Lookup_n-D  BreakpointsForDimension1=ATQR_EL1FEDUTqIncSR_Y_pct  BreakpointsForDimension2=ATQR_EL1FEDUTqIncSR_X_rpm  Table=MTQR_EL1FEDUTqIncSR_Z_Nm  ExtrapMethod=Clip  InternalRulePriority=Speed  RndMeth=Simplest  InputSameDT=on
      settings: InputPortMap=u0,u1
  VTQR_EL1FEDUTqIncSR_Nm : Outport
  wires:
  VTQD_TqTargetShaftSpd_rpm/1 -> MTQR_EL1FEDUTqIncSR_Z_Nm/2
  MTQR_EL1FEDUTqIncSR_Z_Nm/1 -> VTQR_EL1FEDUTqIncSR_Nm/1
  VDHP_ActAPSPosn_pct/1 -> MTQR_EL1FEDUTqIncSR_Z_Nm/1

== system tqr/TQR/Determine Torque Request/TorqueArbitrament/TorqueSmooth/Front wheel rate limit determination/VTQR_ECOFEDURateLimitInc_Nm/LV1 ==
  VDHP_ActAPSPosn_pct : Inport
  VTQD_TqTargetShaftSpd_rpm : Inport  Port=2
  VTQR_EcoTqFrIncGain_c : Inport  Port=3
  Action Port : ActionPort
  MTQR_EL1FEDUTqIncSR_Z_Nm : Lookup_n-D  BreakpointsForDimension1=ATQR_EL1FEDUTqIncSR_Y_pct  BreakpointsForDimension2=ATQR_EL1FEDUTqIncSR_X_rpm  Table=MTQR_EL1FEDUTqIncSR_Z_Nm  ExtrapMethod=Clip  InternalRulePriority=Speed  RndMeth=Simplest  InputSameDT=on
      settings: InputPortMap=u0,u1
  Product : Product
  VTQR_EL1FEDUTqIncSR_Nm : Outport
  wires:
  VDHP_ActAPSPosn_pct/1 -> MTQR_EL1FEDUTqIncSR_Z_Nm/1
  VTQD_TqTargetShaftSpd_rpm/1 -> MTQR_EL1FEDUTqIncSR_Z_Nm/2
  MTQR_EL1FEDUTqIncSR_Z_Nm/1 -> Product/1
  Product/1 -> VTQR_EL1FEDUTqIncSR_Nm/1
  VTQR_EcoTqFrIncGain_c/1 -> Product/2

== system tqr/TQR/Determine Torque Request/TorqueArbitrament/TorqueSmooth/Front wheel rate limit determination/VTQR_ECOFEDURateLimitInc_Nm/LV2 ==
  VDHP_ActAPSPosn_pct : Inport
  VTQD_TqTargetShaftSpd_rpm : Inport  Port=2
  VTQR_EcoTqFrIncGain_c : Inport  Port=3
  Action Port : ActionPort
  MTQR_EL2FEDUTqIncSR_Z_Nm : Lookup_n-D  BreakpointsForDimension1=ATQR_EL1FEDUTqIncSR_Y_pct  BreakpointsForDimension2=ATQR_EL1FEDUTqIncSR_X_rpm  Table=MTQR_EL2FEDUTqIncSR_Z_Nm  ExtrapMethod=Clip  InternalRulePriority=Speed  RndMeth=Simplest  InputSameDT=on
      settings: InputPortMap=u0,u1
  Product : Product
  VTQR_EL2FEDUTqIncSR_Nm : Outport
  wires:
  VDHP_ActAPSPosn_pct/1 -> MTQR_EL2FEDUTqIncSR_Z_Nm/1
  VTQD_TqTargetShaftSpd_rpm/1 -> MTQR_EL2FEDUTqIncSR_Z_Nm/2
  VTQR_EcoTqFrIncGain_c/1 -> Product/2
  MTQR_EL2FEDUTqIncSR_Z_Nm/1 -> Product/1
  Product/1 -> VTQR_EL2FEDUTqIncSR_Nm/1

== system tqr/TQR/Determine Torque Request/TorqueArbitrament/TorqueSmooth/Front wheel rate limit determination/VTQR_ECOFEDURateLimitInc_Nm/LV3 ==
  VDHP_ActAPSPosn_pct : Inport
  VTQD_TqTargetShaftSpd_rpm : Inport  Port=2
  VTQR_EcoTqFrIncGain_c : Inport  Port=3
  Action Port : ActionPort
  MTQR_EL3FEDUTqIncSR_Z_Nm : Lookup_n-D  BreakpointsForDimension1=ATQR_EL1FEDUTqIncSR_Y_pct  BreakpointsForDimension2=ATQR_EL1FEDUTqIncSR_X_rpm  Table=MTQR_EL3FEDUTqIncSR_Z_Nm  ExtrapMethod=Clip  InternalRulePriority=Speed  RndMeth=Simplest  InputSameDT=on
      settings: InputPortMap=u0,u1
  Product : Product
  VTQR_EL3FEDUTqIncSR_Nm : Outport
  wires:
  VDHP_ActAPSPosn_pct/1 -> MTQR_EL3FEDUTqIncSR_Z_Nm/1
  VTQD_TqTargetShaftSpd_rpm/1 -> MTQR_EL3FEDUTqIncSR_Z_Nm/2
  VTQR_EcoTqFrIncGain_c/1 -> Product/2
  MTQR_EL3FEDUTqIncSR_Z_Nm/1 -> Product/1
  Product/1 -> VTQR_EL3FEDUTqIncSR_Nm/1

== system tqr/TQR/Determine Torque Request/TorqueArbitrament/TorqueSmooth/Front wheel rate limit determination/VTQR_ECOFEDURateLimitInc_Nm/LV4 ==
  VDHP_ActAPSPosn_pct : Inport
  VTQD_TqTargetShaftSpd_rpm : Inport  Port=2
  VTQR_EcoTqFrIncGain_c : Inport  Port=3
  Action Port : ActionPort
  MTQR_EL4FEDUTqIncSR_Z_Nm : Lookup_n-D  BreakpointsForDimension1=ATQR_EL1FEDUTqIncSR_Y_pct  BreakpointsForDimension2=ATQR_EL1FEDUTqIncSR_X_rpm  Table=MTQR_EL4FEDUTqIncSR_Z_Nm  ExtrapMethod=Clip  InternalRulePriority=Speed  RndMeth=Simplest  InputSameDT=on
      settings: InputPortMap=u0,u1
  Product : Product
  VTQR_EL4FEDUTqIncSR_Nm : Outport
  wires:
  VDHP_ActAPSPosn_pct/1 -> MTQR_EL4FEDUTqIncSR_Z_Nm/1
  VTQD_TqTargetShaftSpd_rpm/1 -> MTQR_EL4FEDUTqIncSR_Z_Nm/2
  VTQR_EcoTqFrIncGain_c/1 -> Product/2
  MTQR_EL4FEDUTqIncSR_Z_Nm/1 -> Product/1
  Product/1 -> VTQR_EL4FEDUTqIncSR_Nm/1

== system tqr/TQR/Determine Torque Request/TorqueArbitrament/TorqueSmooth/Front wheel rate limit determination/VTQR_ECOFEDURateLimitInc_Nm/LV5 ==
  VDHP_ActAPSPosn_pct : Inport
  VTQD_TqTargetShaftSpd_rpm : Inport  Port=2
  VTQR_EcoTqFrIncGain_c : Inport  Port=3
  Action Port : ActionPort
  MTQR_EL5FEDUTqIncSR_Z_Nm : Lookup_n-D  BreakpointsForDimension1=ATQR_EL1FEDUTqIncSR_Y_pct  BreakpointsForDimension2=ATQR_EL1FEDUTqIncSR_X_rpm  Table=MTQR_EL5FEDUTqIncSR_Z_Nm  ExtrapMethod=Clip  InternalRulePriority=Speed  RndMeth=Simplest  InputSameDT=on
      settings: InputPortMap=u0,u1
  Product : Product
  VTQR_EL5FEDUTqIncSR_Nm : Outport
  wires:
  VDHP_ActAPSPosn_pct/1 -> MTQR_EL5FEDUTqIncSR_Z_Nm/1
  VTQD_TqTargetShaftSpd_rpm/1 -> MTQR_EL5FEDUTqIncSR_Z_Nm/2
  VTQR_EcoTqFrIncGain_c/1 -> Product/2
  MTQR_EL5FEDUTqIncSR_Z_Nm/1 -> Product/1
  Product/1 -> VTQR_EL5FEDUTqIncSR_Nm/1

== system tqr/TQR/Determine Torque Request/TorqueArbitrament/TorqueSmooth/Front wheel rate limit determination/VTQR_ECOFEDURateLimitInc_Nm/OPD ==
  VDHP_ActAPSPosn_pct : Inport
  VTQD_TqTargetShaftSpd_rpm : Inport  Port=2
  VTQR_EcoTqFrIncGain_c : Inport  Port=3
  Action Port : ActionPort
  MTQR_EOPDFEDUTqIncSR_Z_Nm : Lookup_n-D  BreakpointsForDimension1=ATQR_EL1FEDUTqIncSR_Y_pct  BreakpointsForDimension2=ATQR_EL1FEDUTqIncSR_X_rpm  Table=MTQR_EOPDFEDUTqIncSR_Z_Nm  ExtrapMethod=Clip  InternalRulePriority=Speed  RndMeth=Simplest  InputSameDT=on
      settings: InputPortMap=u0,u1
  Product : Product
  VTQR_EOPDFEDUTqIncSR_Nm : Outport
  wires:
  VDHP_ActAPSPosn_pct/1 -> MTQR_EOPDFEDUTqIncSR_Z_Nm/1
  VTQD_TqTargetShaftSpd_rpm/1 -> MTQR_EOPDFEDUTqIncSR_Z_Nm/2
  VTQR_EcoTqFrIncGain_c/1 -> Product/2
  MTQR_EOPDFEDUTqIncSR_Z_Nm/1 -> Product/1
  Product/1 -> VTQR_EOPDFEDUTqIncSR_Nm/1

== system tqr/TQR/Determine Torque Request/TorqueArbitrament/TorqueSmooth/Front wheel rate limit determination/VTQR_NORMALFEDURateLimitDec_Nm/Invalid ==
  VTQR_FEDUWhlTqReqSmoothDelay_Nm : Inport
  VTQD_TqTargetShaftSpd_rpm : Inport  Port=2
  Action Port : ActionPort
  MTQR_NL1FEDUTqDecSR_Z_Nm : Lookup_n-D  BreakpointsForDimension1=ATQR_NL1FEDUTqDecSR_Y_Nm  BreakpointsForDimension2=ATQR_NL1FEDUTqIncSR_X_rpm  Table=MTQR_NL1FEDUTqDecSR_Z_Nm  ExtrapMethod=Clip  InternalRulePriority=Speed  RndMeth=Simplest  InputSameDT=on
      settings: InputPortMap=u0,u1
  VTQR_NL1FEDUTqDecSR_Nm : Outport
  wires:
  VTQD_TqTargetShaftSpd_rpm/1 -> MTQR_NL1FEDUTqDecSR_Z_Nm/2
  MTQR_NL1FEDUTqDecSR_Z_Nm/1 -> VTQR_NL1FEDUTqDecSR_Nm/1
  VTQR_FEDUWhlTqReqSmoothDelay_Nm/1 -> MTQR_NL1FEDUTqDecSR_Z_Nm/1

== system tqr/TQR/Determine Torque Request/TorqueArbitrament/TorqueSmooth/Front wheel rate limit determination/VTQR_NORMALFEDURateLimitDec_Nm/LV1 ==
  VTQR_FEDUWhlTqReqSmoothDelay_Nm : Inport
  VTQD_TqTargetShaftSpd_rpm : Inport  Port=2
  Action Port : ActionPort
  MTQR_NL1FEDUTqDecSR_Z_Nm : Lookup_n-D  BreakpointsForDimension1=ATQR_NL1FEDUTqDecSR_Y_Nm  BreakpointsForDimension2=ATQR_NL1FEDUTqIncSR_X_rpm  Table=MTQR_NL1FEDUTqDecSR_Z_Nm  ExtrapMethod=Clip  InternalRulePriority=Speed  RndMeth=Simplest  InputSameDT=on
      settings: InputPortMap=u0,u1
  VTQR_NL1FEDUTqDecSR_Nm : Outport
  wires:
  VTQR_FEDUWhlTqReqSmoothDelay_Nm/1 -> MTQR_NL1FEDUTqDecSR_Z_Nm/1
  MTQR_NL1FEDUTqDecSR_Z_Nm/1 -> VTQR_NL1FEDUTqDecSR_Nm/1
  VTQD_TqTargetShaftSpd_rpm/1 -> MTQR_NL1FEDUTqDecSR_Z_Nm/2

== system tqr/TQR/Determine Torque Request/TorqueArbitrament/TorqueSmooth/Front wheel rate limit determination/VTQR_NORMALFEDURateLimitDec_Nm/LV2 ==
  VTQR_FEDUWhlTqReqSmoothDelay_Nm : Inport
  VTQD_TqTargetShaftSpd_rpm : Inport  Port=2
  Action Port : ActionPort
  MTQR_NL2FEDUTqDecSR_Z_Nm : Lookup_n-D  BreakpointsForDimension1=ATQR_NL1FEDUTqDecSR_Y_Nm  BreakpointsForDimension2=ATQR_NL1FEDUTqIncSR_X_rpm  Table=MTQR_NL2FEDUTqDecSR_Z_Nm  ExtrapMethod=Clip  InternalRulePriority=Speed  RndMeth=Simplest  InputSameDT=on
      settings: InputPortMap=u0,u1
  VTQR_NL2FEDUTqDecSR_Nm : Outport
  wires:
  MTQR_NL2FEDUTqDecSR_Z_Nm/1 -> VTQR_NL2FEDUTqDecSR_Nm/1
  VTQR_FEDUWhlTqReqSmoothDelay_Nm/1 -> MTQR_NL2FEDUTqDecSR_Z_Nm/1
  VTQD_TqTargetShaftSpd_rpm/1 -> MTQR_NL2FEDUTqDecSR_Z_Nm/2

== system tqr/TQR/Determine Torque Request/TorqueArbitrament/TorqueSmooth/Front wheel rate limit determination/VTQR_NORMALFEDURateLimitDec_Nm/LV3 ==
  VTQR_FEDUWhlTqReqSmoothDelay_Nm : Inport
  VTQD_TqTargetShaftSpd_rpm : Inport  Port=2
  Action Port : ActionPort
  MTQR_NL3FEDUTqDecSR_Z_Nm : Lookup_n-D  BreakpointsForDimension1=ATQR_NL1FEDUTqDecSR_Y_Nm  BreakpointsForDimension2=ATQR_NL1FEDUTqIncSR_X_rpm  Table=MTQR_NL3FEDUTqDecSR_Z_Nm  ExtrapMethod=Clip  InternalRulePriority=Speed  RndMeth=Simplest  InputSameDT=on
      settings: InputPortMap=u0,u1
  VTQR_NL3FEDUTqDecSR_Nm : Outport
  wires:
  VTQR_FEDUWhlTqReqSmoothDelay_Nm/1 -> MTQR_NL3FEDUTqDecSR_Z_Nm/1
  VTQD_TqTargetShaftSpd_rpm/1 -> MTQR_NL3FEDUTqDecSR_Z_Nm/2
  MTQR_NL3FEDUTqDecSR_Z_Nm/1 -> VTQR_NL3FEDUTqDecSR_Nm/1

== system tqr/TQR/Determine Torque Request/TorqueArbitrament/TorqueSmooth/Front wheel rate limit determination/VTQR_NORMALFEDURateLimitDec_Nm/LV4 ==
  VTQR_FEDUWhlTqReqSmoothDelay_Nm : Inport
  VTQD_TqTargetShaftSpd_rpm : Inport  Port=2
  Action Port : ActionPort
  MTQR_NL4FEDUTqDecSR_Z_Nm : Lookup_n-D  BreakpointsForDimension1=ATQR_NL1FEDUTqDecSR_Y_Nm  BreakpointsForDimension2=ATQR_NL1FEDUTqIncSR_X_rpm  Table=MTQR_NL4FEDUTqDecSR_Z_Nm  ExtrapMethod=Clip  InternalRulePriority=Speed  RndMeth=Simplest  InputSameDT=on
      settings: InputPortMap=u0,u1
  VTQR_NL4FEDUTqDecSR_Nm : Outport
  wires:
  VTQR_FEDUWhlTqReqSmoothDelay_Nm/1 -> MTQR_NL4FEDUTqDecSR_Z_Nm/1
  VTQD_TqTargetShaftSpd_rpm/1 -> MTQR_NL4FEDUTqDecSR_Z_Nm/2
  MTQR_NL4FEDUTqDecSR_Z_Nm/1 -> VTQR_NL4FEDUTqDecSR_Nm/1

== system tqr/TQR/Determine Torque Request/TorqueArbitrament/TorqueSmooth/Front wheel rate limit determination/VTQR_NORMALFEDURateLimitDec_Nm/LV5 ==
  VTQR_FEDUWhlTqReqSmoothDelay_Nm : Inport
  VTQD_TqTargetShaftSpd_rpm : Inport  Port=2
  Action Port : ActionPort
  MTQR_NL5FEDUTqDecSR_Z_Nm : Lookup_n-D  BreakpointsForDimension1=ATQR_NL1FEDUTqDecSR_Y_Nm  BreakpointsForDimension2=ATQR_NL1FEDUTqIncSR_X_rpm  Table=MTQR_NL5FEDUTqDecSR_Z_Nm  ExtrapMethod=Clip  InternalRulePriority=Speed  RndMeth=Simplest  InputSameDT=on
      settings: InputPortMap=u0,u1
  VTQR_NL5FEDUTqIDecSR_Nm : Outport
  wires:
  VTQR_FEDUWhlTqReqSmoothDelay_Nm/1 -> MTQR_NL5FEDUTqDecSR_Z_Nm/1
  VTQD_TqTargetShaftSpd_rpm/1 -> MTQR_NL5FEDUTqDecSR_Z_Nm/2
  MTQR_NL5FEDUTqDecSR_Z_Nm/1 -> VTQR_NL5FEDUTqIDecSR_Nm/1

== system tqr/TQR/Determine Torque Request/TorqueArbitrament/TorqueSmooth/Front wheel rate limit determination/VTQR_NORMALFEDURateLimitDec_Nm/OPD ==
  VTQR_FEDUWhlTqReqSmoothDelay_Nm : Inport
  VTQD_TqTargetShaftSpd_rpm : Inport  Port=2
  Action Port : ActionPort
  MTQR_NOPDFEDUTqDecSR_Z_Nm : Lookup_n-D  BreakpointsForDimension1=ATQR_NL1FEDUTqDecSR_Y_Nm  BreakpointsForDimension2=ATQR_NL1FEDUTqIncSR_X_rpm  Table=MTQR_NOPDFEDUTqDecSR_Z_Nm  ExtrapMethod=Clip  InternalRulePriority=Speed  RndMeth=Simplest  InputSameDT=on
      settings: InputPortMap=u0,u1
  VTQR_NOPDFEDUTqDecSR_Nm : Outport
  wires:
  VTQR_FEDUWhlTqReqSmoothDelay_Nm/1 -> MTQR_NOPDFEDUTqDecSR_Z_Nm/1
  VTQD_TqTargetShaftSpd_rpm/1 -> MTQR_NOPDFEDUTqDecSR_Z_Nm/2
  MTQR_NOPDFEDUTqDecSR_Z_Nm/1 -> VTQR_NOPDFEDUTqDecSR_Nm/1

== system tqr/TQR/Determine Torque Request/TorqueArbitrament/TorqueSmooth/Front wheel rate limit determination/VTQR_NORMALFEDURateLimitInc_Nm/Invalid ==
  VDHP_ActAPSPosn_pct : Inport
  VTQD_TqTargetShaftSpd_rpm : Inport  Port=2
  Action Port : ActionPort
  MTQR_NL1FEDUTqIncSR_Z_Nm : Lookup_n-D  BreakpointsForDimension1=ATQR_NL1FEDUTqIncSR_Y_pct  BreakpointsForDimension2=ATQR_NL1FEDUTqIncSR_X_rpm  Table=MTQR_NL1FEDUTqIncSR_Z_Nm  ExtrapMethod=Clip  InternalRulePriority=Speed  RndMeth=Simplest  InputSameDT=on
      settings: InputPortMap=u0,u1
  VTQR_NL1FEDUTqIncSR_Nm : Outport
  wires:
  VTQD_TqTargetShaftSpd_rpm/1 -> MTQR_NL1FEDUTqIncSR_Z_Nm/2
  VDHP_ActAPSPosn_pct/1 -> MTQR_NL1FEDUTqIncSR_Z_Nm/1
  MTQR_NL1FEDUTqIncSR_Z_Nm/1 -> VTQR_NL1FEDUTqIncSR_Nm/1

== system tqr/TQR/Determine Torque Request/TorqueArbitrament/TorqueSmooth/Front wheel rate limit determination/VTQR_NORMALFEDURateLimitInc_Nm/LV1 ==
  VDHP_ActAPSPosn_pct : Inport
  VTQD_TqTargetShaftSpd_rpm : Inport  Port=2
  Action Port : ActionPort
  MTQR_NL1FEDUTqIncSR_Z_Nm : Lookup_n-D  BreakpointsForDimension1=ATQR_NL1FEDUTqIncSR_Y_pct  BreakpointsForDimension2=ATQR_NL1FEDUTqIncSR_X_rpm  Table=MTQR_NL1FEDUTqIncSR_Z_Nm  ExtrapMethod=Clip  InternalRulePriority=Speed  RndMeth=Simplest  InputSameDT=on
      settings: InputPortMap=u0,u1
  VTQR_NL1FEDUTqIncSR_Nm : Outport
  wires:
  VDHP_ActAPSPosn_pct/1 -> MTQR_NL1FEDUTqIncSR_Z_Nm/1
  MTQR_NL1FEDUTqIncSR_Z_Nm/1 -> VTQR_NL1FEDUTqIncSR_Nm/1
  VTQD_TqTargetShaftSpd_rpm/1 -> MTQR_NL1FEDUTqIncSR_Z_Nm/2

== system tqr/TQR/Determine Torque Request/TorqueArbitrament/TorqueSmooth/Front wheel rate limit determination/VTQR_NORMALFEDURateLimitInc_Nm/LV2 ==
  VDHP_ActAPSPosn_pct : Inport
  VTQD_TqTargetShaftSpd_rpm : Inport  Port=2
  VTQR_NormalTqFrIncGain_c : Inport  Port=3
  Action Port : ActionPort
  MTQR_NL2FEDUTqIncSR_Z_Nm : Lookup_n-D  BreakpointsForDimension1=ATQR_NL1FEDUTqIncSR_Y_pct  BreakpointsForDimension2=ATQR_NL1FEDUTqIncSR_X_rpm  Table=MTQR_NL2FEDUTqIncSR_Z_Nm  ExtrapMethod=Clip  InternalRulePriority=Speed  RndMeth=Simplest  InputSameDT=on
      settings: InputPortMap=u0,u1
  Product : Product
  VTQR_NL2FEDUTqIncSR_Nm : Outport
  wires:
  VDHP_ActAPSPosn_pct/1 -> MTQR_NL2FEDUTqIncSR_Z_Nm/1
  VTQD_TqTargetShaftSpd_rpm/1 -> MTQR_NL2FEDUTqIncSR_Z_Nm/2
  MTQR_NL2FEDUTqIncSR_Z_Nm/1 -> Product/1
  Product/1 -> VTQR_NL2FEDUTqIncSR_Nm/1
  VTQR_NormalTqFrIncGain_c/1 -> Product/2

== system tqr/TQR/Determine Torque Request/TorqueArbitrament/TorqueSmooth/Front wheel rate limit determination/VTQR_NORMALFEDURateLimitInc_Nm/LV3 ==
  VDHP_ActAPSPosn_pct : Inport
  VTQD_TqTargetShaftSpd_rpm : Inport  Port=2
  VTQR_NormalTqFrIncGain_c : Inport  Port=3
  Action Port : ActionPort
  MTQR_NL3FEDUTqIncSR_Z_Nm : Lookup_n-D  BreakpointsForDimension1=ATQR_NL1FEDUTqIncSR_Y_pct  BreakpointsForDimension2=ATQR_NL1FEDUTqIncSR_X_rpm  Table=MTQR_NL3FEDUTqIncSR_Z_Nm  ExtrapMethod=Clip  InternalRulePriority=Speed  RndMeth=Simplest  InputSameDT=on
      settings: InputPortMap=u0,u1
  Product : Product
  VTQR_NL3FEDUTqIncSR_Nm : Outport
  wires:
  VDHP_ActAPSPosn_pct/1 -> MTQR_NL3FEDUTqIncSR_Z_Nm/1
  VTQD_TqTargetShaftSpd_rpm/1 -> MTQR_NL3FEDUTqIncSR_Z_Nm/2
  MTQR_NL3FEDUTqIncSR_Z_Nm/1 -> Product/1
  Product/1 -> VTQR_NL3FEDUTqIncSR_Nm/1
  VTQR_NormalTqFrIncGain_c/1 -> Product/2

== system tqr/TQR/Determine Torque Request/TorqueArbitrament/TorqueSmooth/Front wheel rate limit determination/VTQR_NORMALFEDURateLimitInc_Nm/LV4 ==
  VDHP_ActAPSPosn_pct : Inport
  VTQD_TqTargetShaftSpd_rpm : Inport  Port=2
  VTQR_NormalTqFrIncGain_c : Inport  Port=3
  Action Port : ActionPort
  MTQR_NL4FEDUTqIncSR_Z_Nm : Lookup_n-D  BreakpointsForDimension1=ATQR_NL1FEDUTqIncSR_Y_pct  BreakpointsForDimension2=ATQR_NL1FEDUTqIncSR_X_rpm  Table=MTQR_NL4FEDUTqIncSR_Z_Nm  ExtrapMethod=Clip  InternalRulePriority=Speed  RndMeth=Simplest  InputSameDT=on
      settings: InputPortMap=u0,u1
  Product : Product
  VTQR_NL4FEDUTqIncSR_Nm : Outport
  wires:
  VDHP_ActAPSPosn_pct/1 -> MTQR_NL4FEDUTqIncSR_Z_Nm/1
  VTQD_TqTargetShaftSpd_rpm/1 -> MTQR_NL4FEDUTqIncSR_Z_Nm/2
  VTQR_NormalTqFrIncGain_c/1 -> Product/2
  MTQR_NL4FEDUTqIncSR_Z_Nm/1 -> Product/1
  Product/1 -> VTQR_NL4FEDUTqIncSR_Nm/1

== system tqr/TQR/Determine Torque Request/TorqueArbitrament/TorqueSmooth/Front wheel rate limit determination/VTQR_NORMALFEDURateLimitInc_Nm/LV5 ==
  VDHP_ActAPSPosn_pct : Inport
  VTQD_TqTargetShaftSpd_rpm : Inport  Port=2
  VTQR_NormalTqFrIncGain_c : Inport  Port=3
  Action Port : ActionPort
  MTQR_NL5FEDUTqIncSR_Z_Nm : Lookup_n-D  BreakpointsForDimension1=ATQR_NL1FEDUTqIncSR_Y_pct  BreakpointsForDimension2=ATQR_NL1FEDUTqIncSR_X_rpm  Table=MTQR_NL5FEDUTqIncSR_Z_Nm  ExtrapMethod=Clip  InternalRulePriority=Speed  RndMeth=Simplest  InputSameDT=on
      settings: InputPortMap=u0,u1
  Product : Product
  VTQR_NL5FEDUTqIncSR_Nm : Outport
  wires:
  VDHP_ActAPSPosn_pct/1 -> MTQR_NL5FEDUTqIncSR_Z_Nm/1
  VTQD_TqTargetShaftSpd_rpm/1 -> MTQR_NL5FEDUTqIncSR_Z_Nm/2
  VTQR_NormalTqFrIncGain_c/1 -> Product/2
  MTQR_NL5FEDUTqIncSR_Z_Nm/1 -> Product/1
  Product/1 -> VTQR_NL5FEDUTqIncSR_Nm/1

== system tqr/TQR/Determine Torque Request/TorqueArbitrament/TorqueSmooth/Front wheel rate limit determination/VTQR_NORMALFEDURateLimitInc_Nm/OPD ==
  VDHP_ActAPSPosn_pct : Inport
  VTQD_TqTargetShaftSpd_rpm : Inport  Port=2
  VTQR_NormalTqFrIncGain_c : Inport  Port=3
  Action Port : ActionPort
  MTQR_NOPDFEDUTqIncSR_Z_Nm : Lookup_n-D  BreakpointsForDimension1=ATQR_NL1FEDUTqIncSR_Y_pct  BreakpointsForDimension2=ATQR_NL1FEDUTqIncSR_X_rpm  Table=MTQR_NOPDFEDUTqIncSR_Z_Nm  ExtrapMethod=Clip  InternalRulePriority=Speed  RndMeth=Simplest  InputSameDT=on
      settings: InputPortMap=u0,u1
  Product : Product
  VTQR_NOPDFEDUTqIncSR_Nm : Outport
  wires:
  VDHP_ActAPSPosn_pct/1 -> MTQR_NOPDFEDUTqIncSR_Z_Nm/1
  VTQD_TqTargetShaftSpd_rpm/1 -> MTQR_NOPDFEDUTqIncSR_Z_Nm/2
  VTQR_NormalTqFrIncGain_c/1 -> Product/2
  MTQR_NOPDFEDUTqIncSR_Z_Nm/1 -> Product/1
  Product/1 -> VTQR_NOPDFEDUTqIncSR_Nm/1

== system tqr/TQR/Determine Torque Request/TorqueArbitrament/TorqueSmooth/Front wheel rate limit determination/VTQR_SPORTFEDURateLimitDec_Nm/Invalid ==
  VTQR_FEDUWhlTqReqSmoothDelay_Nm : Inport
  VTQD_TqTargetShaftSpd_rpm : Inport  Port=2
  Action Port : ActionPort
  MTQR_SL1FEDUTqDecSR_Z_Nm : Lookup_n-D  BreakpointsForDimension1=ATQR_SL1FEDUTqDecSR_Y_Nm  BreakpointsForDimension2=ATQR_SL1FEDUTqIncSR_X_rpm  Table=MTQR_SL1FEDUTqDecSR_Z_Nm  ExtrapMethod=Clip  InternalRulePriority=Speed  RndMeth=Simplest  InputSameDT=on
      settings: InputPortMap=u0,u1
  VTQR_SL1FEDUTqDecSR_Nm : Outport
  wires:
  VTQD_TqTargetShaftSpd_rpm/1 -> MTQR_SL1FEDUTqDecSR_Z_Nm/2
  MTQR_SL1FEDUTqDecSR_Z_Nm/1 -> VTQR_SL1FEDUTqDecSR_Nm/1
  VTQR_FEDUWhlTqReqSmoothDelay_Nm/1 -> MTQR_SL1FEDUTqDecSR_Z_Nm/1

== system tqr/TQR/Determine Torque Request/TorqueArbitrament/TorqueSmooth/Front wheel rate limit determination/VTQR_SPORTFEDURateLimitDec_Nm/LV1 ==
  VTQR_FEDUWhlTqReqSmoothDelay_Nm : Inport
  VTQD_TqTargetShaftSpd_rpm : Inport  Port=2
  Action Port : ActionPort
  MTQR_SL1FEDUTqDecSR_Z_Nm : Lookup_n-D  BreakpointsForDimension1=ATQR_SL1FEDUTqDecSR_Y_Nm  BreakpointsForDimension2=ATQR_SL1FEDUTqIncSR_X_rpm  Table=MTQR_SL1FEDUTqDecSR_Z_Nm  ExtrapMethod=Clip  InternalRulePriority=Speed  RndMeth=Simplest  InputSameDT=on
      settings: InputPortMap=u0,u1
  VTQR_SL1FEDUTqDecSR_Nm : Outport
  wires:
  VTQR_FEDUWhlTqReqSmoothDelay_Nm/1 -> MTQR_SL1FEDUTqDecSR_Z_Nm/1
  MTQR_SL1FEDUTqDecSR_Z_Nm/1 -> VTQR_SL1FEDUTqDecSR_Nm/1
  VTQD_TqTargetShaftSpd_rpm/1 -> MTQR_SL1FEDUTqDecSR_Z_Nm/2

== system tqr/TQR/Determine Torque Request/TorqueArbitrament/TorqueSmooth/Front wheel rate limit determination/VTQR_SPORTFEDURateLimitDec_Nm/LV2 ==
  VTQR_FEDUWhlTqReqSmoothDelay_Nm : Inport
  VTQD_TqTargetShaftSpd_rpm : Inport  Port=2
  Action Port : ActionPort
  MTQR_SL2FEDUTqDecSR_Z_Nm : Lookup_n-D  BreakpointsForDimension1=ATQR_SL1FEDUTqDecSR_Y_Nm  BreakpointsForDimension2=ATQR_SL1FEDUTqIncSR_X_rpm  Table=MTQR_SL2FEDUTqDecSR_Z_Nm  ExtrapMethod=Clip  InternalRulePriority=Speed  RndMeth=Simplest  InputSameDT=on
      settings: InputPortMap=u0,u1
  VTQR_SL2FEDUTqDecSR_Nm : Outport
  wires:
  MTQR_SL2FEDUTqDecSR_Z_Nm/1 -> VTQR_SL2FEDUTqDecSR_Nm/1
  VTQR_FEDUWhlTqReqSmoothDelay_Nm/1 -> MTQR_SL2FEDUTqDecSR_Z_Nm/1
  VTQD_TqTargetShaftSpd_rpm/1 -> MTQR_SL2FEDUTqDecSR_Z_Nm/2

== system tqr/TQR/Determine Torque Request/TorqueArbitrament/TorqueSmooth/Front wheel rate limit determination/VTQR_SPORTFEDURateLimitDec_Nm/LV3 ==
  VTQR_FEDUWhlTqReqSmoothDelay_Nm : Inport
  VTQD_TqTargetShaftSpd_rpm : Inport  Port=2
  Action Port : ActionPort
  MTQR_SL3FEDUTqDecSR_Z_Nm : Lookup_n-D  BreakpointsForDimension1=ATQR_SL1FEDUTqDecSR_Y_Nm  BreakpointsForDimension2=ATQR_SL1FEDUTqIncSR_X_rpm  Table=MTQR_SL3FEDUTqDecSR_Z_Nm  ExtrapMethod=Clip  InternalRulePriority=Speed  RndMeth=Simplest  InputSameDT=on
      settings: InputPortMap=u0,u1
  VTQR_SL3FEDUTqDecSR_Nm : Outport
  wires:
  VTQR_FEDUWhlTqReqSmoothDelay_Nm/1 -> MTQR_SL3FEDUTqDecSR_Z_Nm/1
  VTQD_TqTargetShaftSpd_rpm/1 -> MTQR_SL3FEDUTqDecSR_Z_Nm/2
  MTQR_SL3FEDUTqDecSR_Z_Nm/1 -> VTQR_SL3FEDUTqDecSR_Nm/1

== system tqr/TQR/Determine Torque Request/TorqueArbitrament/TorqueSmooth/Front wheel rate limit determination/VTQR_SPORTFEDURateLimitDec_Nm/LV4 ==
  VTQR_FEDUWhlTqReqSmoothDelay_Nm : Inport
  VTQD_TqTargetShaftSpd_rpm : Inport  Port=2
  Action Port : ActionPort
  MTQR_SL4FEDUTqDecSR_Z_Nm : Lookup_n-D  BreakpointsForDimension1=ATQR_SL1FEDUTqDecSR_Y_Nm  BreakpointsForDimension2=ATQR_SL1FEDUTqIncSR_X_rpm  Table=MTQR_SL4FEDUTqDecSR_Z_Nm  ExtrapMethod=Clip  InternalRulePriority=Speed  RndMeth=Simplest  InputSameDT=on
      settings: InputPortMap=u0,u1
  VTQR_SL4FEDUTqDecSR_Nm : Outport
  wires:
  VTQR_FEDUWhlTqReqSmoothDelay_Nm/1 -> MTQR_SL4FEDUTqDecSR_Z_Nm/1
  VTQD_TqTargetShaftSpd_rpm/1 -> MTQR_SL4FEDUTqDecSR_Z_Nm/2
  MTQR_SL4FEDUTqDecSR_Z_Nm/1 -> VTQR_SL4FEDUTqDecSR_Nm/1

== system tqr/TQR/Determine Torque Request/TorqueArbitrament/TorqueSmooth/Front wheel rate limit determination/VTQR_SPORTFEDURateLimitDec_Nm/LV5 ==
  VTQR_FEDUWhlTqReqSmoothDelay_Nm : Inport
  VTQD_TqTargetShaftSpd_rpm : Inport  Port=2
  Action Port : ActionPort
  MTQR_SL5FEDUTqDecSR_Z_Nm : Lookup_n-D  BreakpointsForDimension1=ATQR_SL1FEDUTqDecSR_Y_Nm  BreakpointsForDimension2=ATQR_SL1FEDUTqIncSR_X_rpm  Table=MTQR_SL5FEDUTqDecSR_Z_Nm  ExtrapMethod=Clip  InternalRulePriority=Speed  RndMeth=Simplest  InputSameDT=on
      settings: InputPortMap=u0,u1
  VTQR_SL5FEDUTqIDecSR_Nm : Outport
  wires:
  VTQR_FEDUWhlTqReqSmoothDelay_Nm/1 -> MTQR_SL5FEDUTqDecSR_Z_Nm/1
  VTQD_TqTargetShaftSpd_rpm/1 -> MTQR_SL5FEDUTqDecSR_Z_Nm/2
  MTQR_SL5FEDUTqDecSR_Z_Nm/1 -> VTQR_SL5FEDUTqIDecSR_Nm/1

== system tqr/TQR/Determine Torque Request/TorqueArbitrament/TorqueSmooth/Front wheel rate limit determination/VTQR_SPORTFEDURateLimitDec_Nm/OPD ==
  VTQR_FEDUWhlTqReqSmoothDelay_Nm : Inport
  VTQD_TqTargetShaftSpd_rpm : Inport  Port=2
  Action Port : ActionPort
  MTQR_SOPDFEDUTqDecSR_Z_Nm : Lookup_n-D  BreakpointsForDimension1=ATQR_SL1FEDUTqDecSR_Y_Nm  BreakpointsForDimension2=ATQR_SL1FEDUTqIncSR_X_rpm  Table=MTQR_SOPDFEDUTqDecSR_Z_Nm  ExtrapMethod=Clip  InternalRulePriority=Speed  RndMeth=Simplest  InputSameDT=on
      settings: InputPortMap=u0,u1
  VTQR_SOPDFEDUTqDecSR_Nm : Outport
  wires:
  VTQR_FEDUWhlTqReqSmoothDelay_Nm/1 -> MTQR_SOPDFEDUTqDecSR_Z_Nm/1
  VTQD_TqTargetShaftSpd_rpm/1 -> MTQR_SOPDFEDUTqDecSR_Z_Nm/2
  MTQR_SOPDFEDUTqDecSR_Z_Nm/1 -> VTQR_SOPDFEDUTqDecSR_Nm/1

== system tqr/TQR/Determine Torque Request/TorqueArbitrament/TorqueSmooth/Front wheel rate limit determination/VTQR_SPORTFEDURateLimitInc_Nm/Invalid ==
  VDHP_ActAPSPosn_pct : Inport
  VTQD_TqTargetShaftSpd_rpm : Inport  Port=2
  Action Port : ActionPort
  MTQR_SL1FEDUTqIncSR_Z_Nm : Lookup_n-D  BreakpointsForDimension1=ATQR_SL1FEDUTqIncSR_Y_pct  BreakpointsForDimension2=ATQR_SL1FEDUTqIncSR_X_rpm  Table=MTQR_SL1FEDUTqIncSR_Z_Nm  ExtrapMethod=Clip  InternalRulePriority=Speed  RndMeth=Simplest  InputSameDT=on
      settings: InputPortMap=u0,u1
  VTQR_SL1FEDUTqIncSR_Nm : Outport
  wires:
  VDHP_ActAPSPosn_pct/1 -> MTQR_SL1FEDUTqIncSR_Z_Nm/1
  MTQR_SL1FEDUTqIncSR_Z_Nm/1 -> VTQR_SL1FEDUTqIncSR_Nm/1
  VTQD_TqTargetShaftSpd_rpm/1 -> MTQR_SL1FEDUTqIncSR_Z_Nm/2

== system tqr/TQR/Determine Torque Request/TorqueArbitrament/TorqueSmooth/Front wheel rate limit determination/VTQR_SPORTFEDURateLimitInc_Nm/LV1 ==
  VDHP_ActAPSPosn_pct : Inport
  VTQD_TqTargetShaftSpd_rpm : Inport  Port=2
  VTQR_SportTqFrIncGain_c : Inport  Port=3
  Action Port : ActionPort
  MTQR_SL1FEDUTqIncSR_Z_Nm : Lookup_n-D  BreakpointsForDimension1=ATQR_SL1FEDUTqIncSR_Y_pct  BreakpointsForDimension2=ATQR_SL1FEDUTqIncSR_X_rpm  Table=MTQR_SL1FEDUTqIncSR_Z_Nm  ExtrapMethod=Clip  InternalRulePriority=Speed  RndMeth=Simplest  InputSameDT=on
      settings: InputPortMap=u0,u1
  Product : Product
  VTQR_SL1FEDUTqIncSR_Nm : Outport
  wires:
  VTQD_TqTargetShaftSpd_rpm/1 -> MTQR_SL1FEDUTqIncSR_Z_Nm/2
  VDHP_ActAPSPosn_pct/1 -> MTQR_SL1FEDUTqIncSR_Z_Nm/1
  MTQR_SL1FEDUTqIncSR_Z_Nm/1 -> Product/1
  Product/1 -> VTQR_SL1FEDUTqIncSR_Nm/1
  VTQR_SportTqFrIncGain_c/1 -> Product/2

== system tqr/TQR/Determine Torque Request/TorqueArbitrament/TorqueSmooth/Front wheel rate limit determination/VTQR_SPORTFEDURateLimitInc_Nm/LV2 ==
  VDHP_ActAPSPosn_pct : Inport
  VTQD_TqTargetShaftSpd_rpm : Inport  Port=2
  VTQR_SportTqFrIncGain_c : Inport  Port=3
  Action Port : ActionPort
  MTQR_SL2FEDUTqIncSR_Z_Nm : Lookup_n-D  BreakpointsForDimension1=ATQR_SL1FEDUTqIncSR_Y_pct  BreakpointsForDimension2=ATQR_SL1FEDUTqIncSR_X_rpm  Table=MTQR_SL2FEDUTqIncSR_Z_Nm  ExtrapMethod=Clip  InternalRulePriority=Speed  RndMeth=Simplest  InputSameDT=on
      settings: InputPortMap=u0,u1
  Product : Product
  VTQR_SL2FEDUTqIncSR_Nm : Outport
  wires:
  VTQD_TqTargetShaftSpd_rpm/1 -> MTQR_SL2FEDUTqIncSR_Z_Nm/2
  VDHP_ActAPSPosn_pct/1 -> MTQR_SL2FEDUTqIncSR_Z_Nm/1
  VTQR_SportTqFrIncGain_c/1 -> Product/2
  MTQR_SL2FEDUTqIncSR_Z_Nm/1 -> Product/1
  Product/1 -> VTQR_SL2FEDUTqIncSR_Nm/1

== system tqr/TQR/Determine Torque Request/TorqueArbitrament/TorqueSmooth/Front wheel rate limit determination/VTQR_SPORTFEDURateLimitInc_Nm/LV3 ==
  VDHP_ActAPSPosn_pct : Inport
  VTQD_TqTargetShaftSpd_rpm : Inport  Port=2
  VTQR_SportTqFrIncGain_c : Inport  Port=3
  Action Port : ActionPort
  MTQR_SL3FEDUTqIncSR_Z_Nm : Lookup_n-D  BreakpointsForDimension1=ATQR_SL1FEDUTqIncSR_Y_pct  BreakpointsForDimension2=ATQR_SL1FEDUTqIncSR_X_rpm  Table=MTQR_SL3FEDUTqIncSR_Z_Nm  ExtrapMethod=Clip  InternalRulePriority=Speed  RndMeth=Simplest  InputSameDT=on
      settings: InputPortMap=u0,u1
  Product : Product
  VTQR_SL3FEDUTqIncSR_Nm : Outport
  wires:
  VTQD_TqTargetShaftSpd_rpm/1 -> MTQR_SL3FEDUTqIncSR_Z_Nm/2
  VDHP_ActAPSPosn_pct/1 -> MTQR_SL3FEDUTqIncSR_Z_Nm/1
  VTQR_SportTqFrIncGain_c/1 -> Product/2
  MTQR_SL3FEDUTqIncSR_Z_Nm/1 -> Product/1
  Product/1 -> VTQR_SL3FEDUTqIncSR_Nm/1
